simulink model "tut06"  (R2024a)
settings: Solver=VariableStepAuto  StartTime=0.0  StopTime=10.0  RelTol=1e-3
libraries: simulink x1, SignalEditorBlockLib x1
settings Model: Creator=User  LastModifiedBy=User

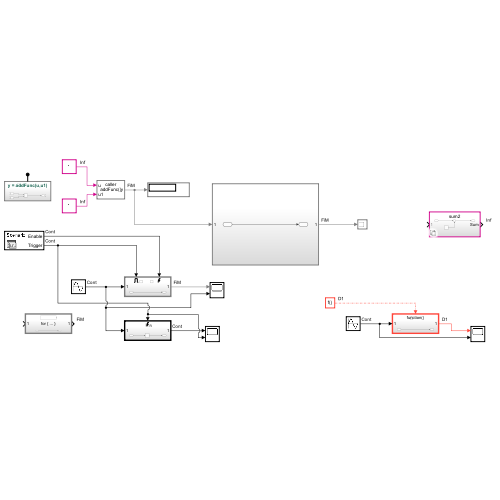
[thumbnail: Simulink's stored preview of the top-level diagram]
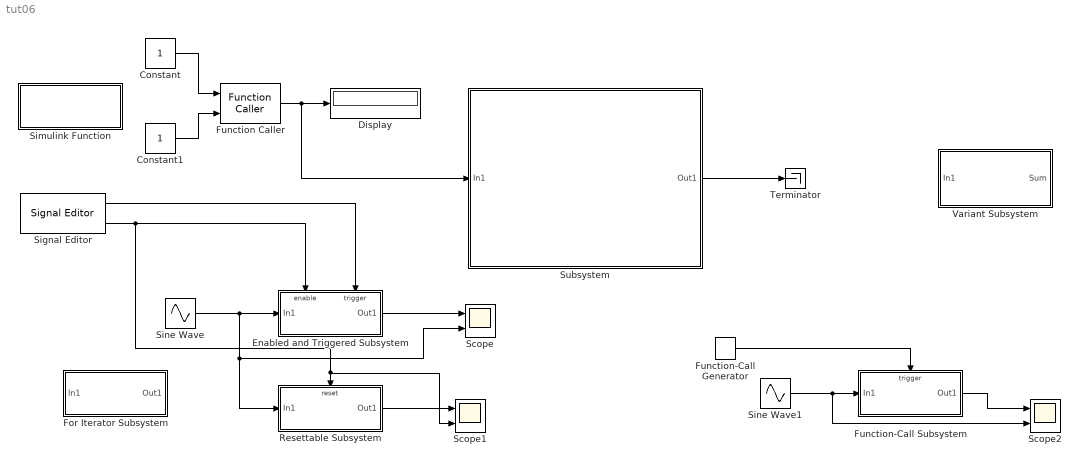
== system tut06 ==
  Constant : Constant
  Constant1 : Constant
  Display : Display
  Enabled and Triggered Subsystem : Subsystem  TreatAsAtomicUnit=on
  For Iterator Subsystem : Subsystem  TreatAsAtomicUnit=on
  Function Caller : FunctionCaller  FunctionPrototype=y = addFunc(u,u1)  InputArgumentSpecifications=<Enter example>  OutputArgumentSpecifications=<Enter example>
  Function-Call Generator : simulink/Ports & Subsystems/Function-Call Generator  sample_time=2e-3  numberOfIterations=1  DisallowWideOutput=off
  Function-Call Subsystem : Subsystem  TreatAsAtomicUnit=on
  Resettable Subsystem : Subsystem  TreatAsAtomicUnit=on
  Scope : Scope  NumInputPorts=2
  Scope1 : Scope  NumInputPorts=2
  Scope2 : Scope  NumInputPorts=2
  Signal Editor : SignalEditorBlockLib/Signal Editor  FileName=D:\ME\Career\04.MBD\Tutorials\SimulinkTut\tut06\untitled.mat  ActiveScenario=Scenario  ActiveSignal=Enable  IsBus=off  OutputBusObjectStr=Bus: BusObject  SampleTime=0  Interpolate=off  ZeroCross=off  OutputAfterFinalValue=Setting to zero  Unit=inherit  PreserveSignalName=on  ApplySigPropsToAllScenarios=on  ApplySigPropsToAllSignals=off
  Simulink Function : Subsystem  TreatAsAtomicUnit=on
  Sine Wave : Sin  SampleTime=0
  Sine Wave1 : Sin  SampleTime=0
  Subsystem : Subsystem
  Terminator : Terminator
  Variant Subsystem : Subsystem  Variant=on
  wires:
  Constant/1 -> Function Caller/1
  Constant1/1 -> Function Caller/2
  Function Caller/1 -> Subsystem/1(In1), Display/1
  Subsystem/1(Out1) -> Terminator/1
  Signal Editor/1 -> Enabled and Triggered Subsystem/Trigger
  Signal Editor/2 -> Scope1/2, Resettable Subsystem/Reset, Enabled and Triggered Subsystem/Enable
  Sine Wave/1 -> Resettable Subsystem/1(In1), Scope/2, Enabled and Triggered Subsystem/1(In1)
  Enabled and Triggered Subsystem/1(Out1) -> Scope/1
  Resettable Subsystem/1(Out1) -> Scope1/1
  Sine Wave1/1 -> Scope2/2, Function-Call Subsystem/1(In1)
  Function-Call Subsystem/1(Out1) -> Scope2/1
  Function-Call Generator/1 -> Function-Call Subsystem/Trigger

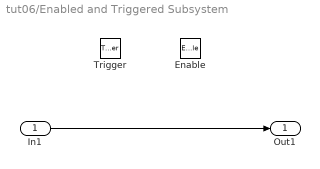
== system tut06/Enabled and Triggered Subsystem ==
  In1 : Inport
  Enable : EnablePort
  Trigger : TriggerPort  VariantControl=(inherit)
  Out1 : Outport
  wires:
  In1/1 -> Out1/1

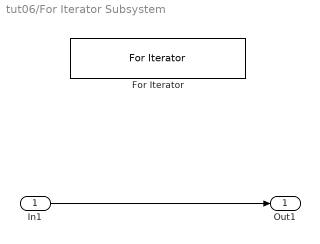
== system tut06/For Iterator Subsystem ==
  In1 : Inport
  For Iterator : ForIterator
  Out1 : Outport
  wires:
  In1/1 -> Out1/1

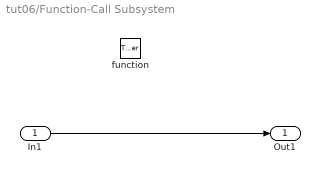
== system tut06/Function-Call Subsystem ==
  In1 : Inport
  function : TriggerPort  TriggerType=function-call  VariantControl=(inherit)
  Out1 : Outport
  wires:
  In1/1 -> Out1/1

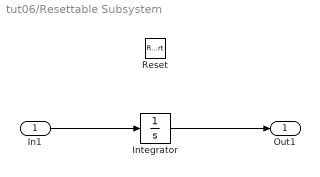
== system tut06/Resettable Subsystem ==
  In1 : Inport
  Reset : ResetPort  DisableCoverage=on
  Integrator : Integrator
  Out1 : Outport
  wires:
  In1/1 -> Integrator/1
  Integrator/1 -> Out1/1

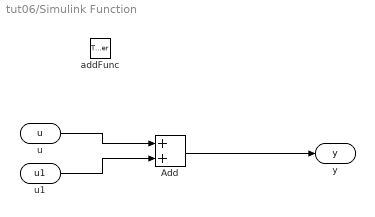
== system tut06/Simulink Function ==
  addFunc : TriggerPort  TriggerType=function-call  IsSimulinkFunction=on  FunctionName=addFunc  FunctionVisibility=scoped  VariantControl=(inherit)
  Add : Sum
  u : ArgIn  DisableCoverage=on  ArgumentName=u
  u1 : ArgIn  DisableCoverage=on  Port=2  ArgumentName=u1
  y : ArgOut  DisableCoverage=on  ArgumentName=y
  wires:
  Add/1 -> y/1
  u/1 -> Add/1
  u1/1 -> Add/2

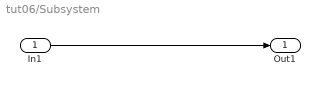
== system tut06/Subsystem ==
  In1 : Inport
  Out1 : Outport
  wires:
  In1/1 -> Out1/1

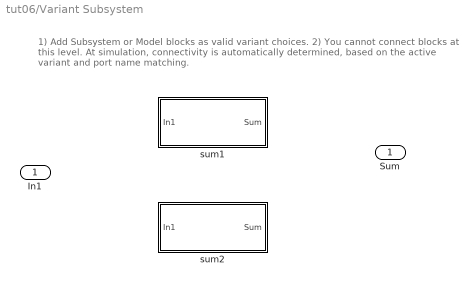
== system tut06/Variant Subsystem ==
  note: 1) Add Subsystem or Model blocks as valid variant choices.
      | 2) You cannot connect blocks at this level. At simulation, connectivity is automatically
      | determined, based on the active variant and port name matching.
  In1 : Inport
  sum1 : Subsystem  VariantControl=Summ==sum1
  sum2 : Subsystem  VariantControl=Summ==sum2
  Sum : Outport

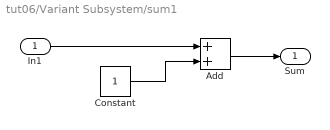
== system tut06/Variant Subsystem/sum1 ==
  In1 : Inport
  Add : Sum
  Constant : Constant
  Sum : Outport
  wires:
  In1/1 -> Add/1
  Constant/1 -> Add/2
  Add/1 -> Sum/1

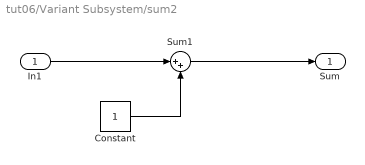
== system tut06/Variant Subsystem/sum2 ==
  In1 : Inport
  Constant : Constant
  Sum1 : Sum  Inputs=|++
  Sum : Outport
  wires:
  In1/1 -> Sum1/1
  Sum1/1 -> Sum/1
  Constant/1 -> Sum1/2
